simulink model "part_C_q17_simulink"  (R2023b)
settings: Solver=VariableStepAuto  StartTime=0.0  StopTime=20  RelTol=1e-3
values from neighbouring files (symbols this model uses):
  a1 = 1.4    [FOUND_full_car.m]
  a2 = 1.47    [FOUND_full_car.m]
  b1 = 0.7    [FOUND_full_car.m]
  b2 = 0.75    [FOUND_full_car.m]
  cf = 5000    [FOUND_full_car.m]
  cr = 5000    [FOUND_full_car.m]
  Ix = 820    [FOUND_full_car.m]
  Iy = 1100    [FOUND_full_car.m]
  kf = 10000    [FOUND_full_car.m]
  kr = 13000    [FOUND_full_car.m]
  ktf = 200000    [FOUND_full_car.m]
  ktr = 200000    [FOUND_full_car.m]
  m = 840    [FOUND_full_car.m]    (also in init_params.m = 240)
  mf = 53    [FOUND_full_car.m]
  mr = 76    [FOUND_full_car.m]
  w = b1+b2    (= 1.45)    [FOUND_full_car.m]    (also in q7.m = 2*pi*f; q8.m = 2*pi*f; roadpr_ISO8608.m = linspace(wmin,wmax,N)')
settings Model: Creator=yusufcagriogut  LastModifiedBy=yusufcagriogut

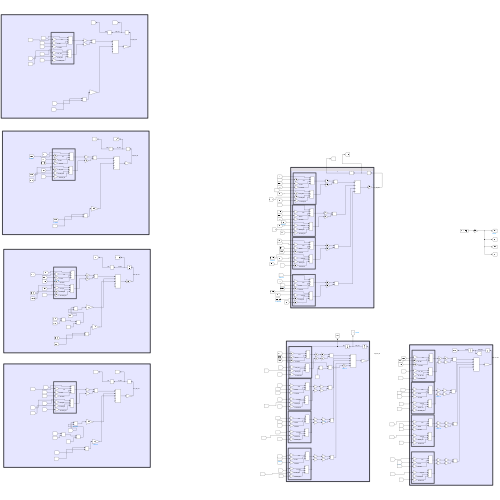
[thumbnail: Simulink's stored preview of the top-level diagram]
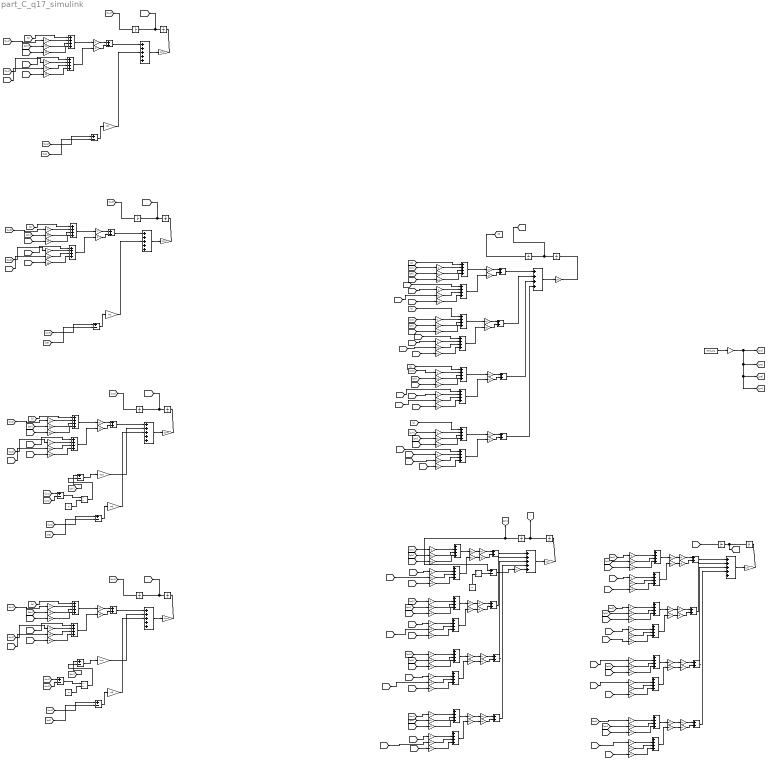
== system part_C_q17_simulink ==
  Add{,10..13,15..17,26,28..30,39,41,47,51} (16 alike) : Sum
  Add{1..9,18..25,31..38,43..46,49..50,53..54} (33 alike) : Sum  Inputs=++++
  Add{14,27,40,42,48,52} (6 alike) : Sum  Inputs=+++++
  Constant : Constant  Value=w
  Constant1 : Constant  Value=w
  Constant2 : Constant  Value=w
  Divide : Product  Inputs=*/
  Divide1 : Product  Inputs=*/
  Divide2 : Product  Inputs=*/
  From Workspace : FromWorkspace  VariableName=road_sig
  Gain : Gain  Gain=-kf
  Gain1 : Gain  Gain=-cf
  Gain{10,13,15,18,35,38,40,43,77,80,82,85,126,130,138,142} (16 alike) : Gain  Gain=-b2
  Gain{29,31,58,74,100} (5 alike) : Gain  Gain=-kr
  Gain{30,32,59,101} (4 alike) : Gain  Gain=-cr
  Gain{4,7,21,24,47,50,60,63,66..67,72..73,89,92,102,105,143,146,153,156} (20 alike) : Gain  Gain=b1
  Gain{5,8,11,14,36,39,61,64,78,81,103,106,127,131,144,147} (16 alike) : Gain  Gain=-a1
  Gain{3,6,9,12,17,20,23,26,37,42,46,49,52,56,62,65,79,84,88,91,94,98,104,107,125,129,137,139,141,145,152,155} (32 alike) : Gain  Gain=-1
  Gain{108..111} (4 alike) : Gain  Gain=a1
  Gain112 : Gain  Gain=-a2
  Gain113 : Gain  Gain=-a2
  Gain{16,19,22,25,41,44,48,51,83,86,90,93,114..115,140,148,154,157} (18 alike) : Gain  Gain=a2
  Gain{53,75,95,116,120} (5 alike) : Gain  Gain=kf
  Gain{54,76,96,117,121} (5 alike) : Gain  Gain=cf
  Gain118 : Gain  Gain=kr/w
  Gain119 : Gain  Gain=-ktf
  Gain122 : Gain  Gain=-kr/w
  Gain123 : Gain  Gain=-ktf
  Gain124 : Gain  Gain=1/mf
  Gain128 : Gain  Gain=1/mf
  Gain{55,97,132,134} (4 alike) : Gain  Gain=kr
  Gain{57,99,133,149} (4 alike) : Gain  Gain=cr
  Gain135 : Gain  Gain=-ktr
  Gain136 : Gain  Gain=1/mr
  Gain150 : Gain  Gain=-ktr
  Gain151 : Gain  Gain=1/mr
  Gain158 : Gain  Gain=0.01
  Gain2 : Gain  Gain=1/m
  Gain27 : Gain  Gain=-kf
  Gain28 : Gain  Gain=-cf
  Gain33 : Gain  Gain=-kf
  Gain34 : Gain  Gain=-cf
  Gain45 : Gain  Gain=1/Ix
  Gain{68..71} (4 alike) : Gain  Gain=b2
  Gain87 : Gain  Gain=1/Iy
  Integrator{,1..13} (14 alike) : Integrator
  Subtract{,1..7,9} (9 alike) : Sum  Inputs=+-
  wires:
  Gain/1 -> Add/1
  Gain1/1 -> Add/2
  Add/1 -> Add1/1
  Add1/1 -> Gain2/1
  Gain2/1 -> Integrator/1  "z_dot_dot"
  Add2/1 -> Gain/1
  Gain3/1 -> Add2/2  "-zu1"
  Gain4/1 -> Add2/3  "b1*phi"
  Gain5/1 -> Add2/4  "-a1*theta"
  Gain6/1 -> Add3/2  "-zu1_dot"
  Gain7/1 -> Add3/3  "b1*phi_dot"
  Gain8/1 -> Add3/4  "-a1*theta_dot"
  Add3/1 -> Gain1/1
  Gain14/1 -> Add5/4  "-a1*theta_dot"
  Gain13/1 -> Add5/3  "-b2*phi_dot"
  Gain12/1 -> Add5/2  "-zu2_dot"
  Gain11/1 -> Add4/4  "-a1*theta"
  Gain10/1 -> Add4/3  "-b2*phi"
  Gain9/1 -> Add4/2  "-zu2"
  Gain20/1 -> Add6/2  "-zu3"
  Gain15/1 -> Add6/3  "-b2*phi"
  Gain16/1 -> Add6/4  "a2*theta"
  Gain17/1 -> Add7/2  "-zu3_dot"
  Gain18/1 -> Add7/3  "-b2*phi_dot"
  Gain19/1 -> Add7/4  "a2*theta_dot"
  Gain21/1 -> Add8/3  "b1*phi"
  Gain25/1 -> Add9/4  "a2*theta_dot"
  Gain26/1 -> Add8/2  "-zu4"
  Gain24/1 -> Add9/3  "b1*phi_dot"
  Gain22/1 -> Add8/4  "a2*theta"
  Gain23/1 -> Add9/2  "-zu4_dot"
  Add5/1 -> Gain28/1
  Add4/1 -> Gain27/1
  Add10/1 -> Add1/2
  Gain28/1 -> Add10/2
  Gain27/1 -> Add10/1
  Gain29/1 -> Add11/1
  Gain30/1 -> Add11/2
  Add11/1 -> Add1/3
  Add6/1 -> Gain29/1
  Add7/1 -> Gain30/1
  Add9/1 -> Gain32/1
  Add8/1 -> Gain31/1
  Gain32/1 -> Add12/2
  Gain31/1 -> Add12/1
  Add12/1 -> Add1/4
  Add15/1 -> Add14/2
  Gain35/1 -> Add20/3  "-b2*phi"
  Add18/1 -> Gain66/1
  Gain58/1 -> Add17/1
  Add23/1 -> Gain70/1
  Gain59/1 -> Add17/2
  Gain62/1 -> Add19/2  "-zu1_dot"
  Gain34/1 -> Add13/2
  Add20/1 -> Gain68/1
  Add25/1 -> Gain73/1
  Add24/1 -> Gain72/1
  Gain57/1 -> Add16/2
  Gain45/1 -> Integrator2/1  "phi_dot_dot"
  Gain51/1 -> Add25/4  "a2*theta_dot"
  Gain56/1 -> Add18/2  "-zu1"
  Gain48/1 -> Add24/4  "a2*theta"
  Gain64/1 -> Add19/4  "-a1*theta_dot"
  Gain33/1 -> Add13/1
  Gain50/1 -> Add25/3  "b1*phi_dot"
  Add21/1 -> Gain69/1
  Gain36/1 -> Add20/4  "-a1*theta"
  Add17/1 -> Add14/4
  Gain38/1 -> Add21/3  "-b2*phi_dot"
  Add14/1 -> Gain45/1
  Gain52/1 -> Add24/2  "-zu4"
  Gain65/1 -> Add20/2  "-zu2"
  Gain49/1 -> Add25/2  "-zu4_dot"
  Gain40/1 -> Add22/3  "-b2*phi"
  Gain63/1 -> Add19/3  "b1*phi_dot"
  Gain60/1 -> Add18/3  "b1*phi"
  Gain47/1 -> Add24/3  "b1*phi"
  Integrator2/1 -> Integrator3/1, [phi_dot]  "phi_dot"
  Add22/1 -> Gain71/1
  Add19/1 -> Gain67/1
  Gain46/1 -> Add22/2  "-zu3"
  Gain61/1 -> Add18/4  "-a1*theta"
  Gain42/1 -> Add23/2  "-zu3_dot"
  Gain37/1 -> Add21/2  "-zu2_dot"
  Gain44/1 -> Add23/4  "a2*theta_dot"
  Add16/1 -> Add14/3
  Gain43/1 -> Add23/3  "-b2*phi_dot"
  Gain41/1 -> Add22/4  "a2*theta"
  Gain39/1 -> Add21/4  "-a1*theta_dot"
  Gain55/1 -> Add16/1
  Add13/1 -> Add14/1
  Gain53/1 -> Add15/1
  Gain54/1 -> Add15/2
  Gain66/1 -> Gain33/1
  Gain67/1 -> Gain34/1
  Integrator3/1 -> [phi], Subtract/1  "phi"
  Gain68/1 -> Gain53/1
  Gain69/1 -> Gain54/1
  Gain70/1 -> Gain57/1
  Gain71/1 -> Gain55/1
  Gain72/1 -> Gain58/1
  Gain73/1 -> Gain59/1
  Gain74/1 -> Add14/5
  Constant/1 -> Divide/2
  Divide/1 -> Subtract/2
  Subtract/1 -> Gain74/1
  Gain114/1 -> Gain100/1
  Gain113/1 -> Gain97/1
  Gain88/1 -> Add35/2  "-zu3"
  Add34/1 -> Gain111/1
  Gain81/1 -> Add34/4  "-a1*theta_dot"
  Gain112/1 -> Gain99/1
  Gain115/1 -> Gain101/1
  Add26/1 -> Add27/1
  Gain82/1 -> Add35/3  "-b2*phi"
  Gain90/1 -> Add37/4  "a2*theta"
  Gain110/1 -> Gain95/1
  Gain96/1 -> Add28/2
  Gain109/1 -> Gain76/1
  Add27/1 -> Gain87/1
  Gain106/1 -> Add32/4  "-a1*theta_dot"
  Gain99/1 -> Add29/2
  Gain87/1 -> Integrator4/1  "theta_dot_dot"
  Add29/1 -> Add27/3
  Gain111/1 -> Gain96/1
  Gain95/1 -> Add28/1
  Add36/1 -> Gain112/1
  Gain89/1 -> Add37/3  "b1*phi"
  Gain77/1 -> Add33/3  "-b2*phi"
  Gain108/1 -> Gain75/1
  Integrator4/1 -> [theta_dot], Integrator5/1  "theta_dot"
  Integrator1/1 -> [z]  "z"
  Gain105/1 -> Add32/3  "b1*phi_dot"
  Add32/1 -> Gain109/1
  Gain84/1 -> Add36/2  "-zu3_dot"
  Add37/1 -> Gain114/1
  Gain85/1 -> Add36/3  "-b2*phi_dot"
  Add35/1 -> Gain113/1
  Gain103/1 -> Add31/4  "-a1*theta"
  Gain79/1 -> Add34/2  "-zu2_dot"
  Add38/1 -> Gain115/1
  Gain97/1 -> Add29/1
  Gain86/1 -> Add36/4  "a2*theta_dot"
  Gain83/1 -> Add35/4  "a2*theta"
  Gain76/1 -> Add26/2
  Gain101/1 -> Add30/2
  Add31/1 -> Gain108/1
  Gain98/1 -> Add31/2  "-zu1"
  Add28/1 -> Add27/2
  Gain94/1 -> Add37/2  "-zu4"
  Gain104/1 -> Add32/2  "-zu1_dot"
  Add33/1 -> Gain110/1
  Gain100/1 -> Add30/1
  Gain93/1 -> Add38/4  "a2*theta_dot"
  Gain107/1 -> Add33/2  "-zu2"
  Gain92/1 -> Add38/3  "b1*phi_dot"
  Add30/1 -> Add27/4
  Gain102/1 -> Add31/3  "b1*phi"
  Gain80/1 -> Add34/3  "-b2*phi_dot"
  Gain78/1 -> Add33/4  "-a1*theta"
  Gain75/1 -> Add26/1
  Gain91/1 -> Add38/2  "-zu4_dot"
  Integrator/1 -> [z_dot], Integrator1/1
  [phi] -> Gain102/1
  Integrator5/1 -> [theta]  "theta"
  [theta] -> Gain103/1
  [theta_dot] -> Gain106/1
  [phi] -> Gain77/1
  [theta] -> Gain78/1
  [phi] -> Gain82/1
  [theta] -> Gain83/1
  [phi] -> Gain89/1
  [theta] -> Gain90/1
  [theta_dot] -> Gain81/1
  [theta_dot] -> Gain86/1
  [theta_dot] -> Gain93/1
  [theta_dot] -> Gain51/1
  [theta] -> Gain48/1
  [phi] -> Gain47/1
  [phi] -> Gain40/1
  [theta] -> Gain41/1
  [phi] -> Gain35/1
  [theta] -> Gain36/1
  [phi] -> Gain60/1
  [theta] -> Gain61/1
  [theta_dot] -> Gain64/1
  [theta_dot] -> Gain39/1
  [theta_dot] -> Gain44/1
  [theta_dot] -> Gain25/1
  [theta_dot] -> Gain19/1
  [theta_dot] -> Gain14/1
  [theta_dot] -> Gain8/1
  [phi] -> Gain4/1
  [theta] -> Gain5/1
  [phi] -> Gain10/1
  [theta] -> Gain11/1
  [phi] -> Gain15/1
  [theta] -> Gain16/1
  [phi] -> Gain21/1
  [theta] -> Gain22/1
  Add39/1 -> Add40/1
  Add45/1 -> Gain117/1
  Add40/1 -> Gain128/1
  Integrator7/1 -> [zu1]  "zu1"
  Gain128/1 -> Integrator6/1  "zu1_dot_dot"
  Add44/1 -> Gain116/1
  Integrator6/1 -> [zu1_dot], Integrator7/1  "zu1_dot"
  Gain144/1 -> Add44/4  "-a1*theta"
  Gain117/1 -> Add39/2
  Gain145/1 -> Add45/2  "-zu1_dot"
  Gain147/1 -> Add45/4  "-a1*theta_dot"
  Gain143/1 -> Add44/3  "b1*phi"
  Gain116/1 -> Add39/1
  [theta_dot] -> Gain147/1
  Gain146/1 -> Add45/3  "b1*phi_dot"
  [phi] -> Gain143/1
  [theta] -> Gain144/1
  Gain139/1 -> Add44/2  "-zu1"
  [z] -> Add44/1
  [zu1] -> Gain139/1
  [z_dot] -> Add45/1
  [zu1] -> Gain145/1
  [phi_dot] -> Gain146/1
  Gain118/1 -> Add40/2
  [phi] -> Subtract1/1
  Constant1/1 -> Divide1/2
  [zu1] -> Subtract2/1
  [zu2] -> Subtract2/2
  Subtract2/1 -> Divide1/1
  Divide1/1 -> Subtract1/2
  Subtract1/1 -> Gain118/1
  [zu1] -> Subtract3/1
  [zr1] -> Subtract3/2
  Subtract3/1 -> Gain119/1
  Gain119/1 -> Add40/3
  [zu2] -> Gain129/1
  Gain127/1 -> Add43/4  "-a1*theta"
  [zu2] -> Subtract5/2
  [zr2] -> Subtract6/2
  Add41/1 -> Add42/1
  Add42/1 -> Gain124/1
  Gain124/1 -> Integrator8/1  "zu2_dot_dot"
  Gain125/1 -> Add43/2  "-zu1"
  [theta] -> Gain127/1
  Integrator9/1 -> [zu2]  "zu2"
  Subtract4/1 -> Gain122/1
  [phi] -> Gain126/1
  Gain130/1 -> Add46/3  "b1*phi_dot"
  [theta_dot] -> Gain131/1
  Gain126/1 -> Add43/3  "b1*phi"
  Gain129/1 -> Add46/2  "-zu1_dot"
  Add43/1 -> Gain120/1
  Gain120/1 -> Add41/1
  Gain131/1 -> Add46/4  "-a1*theta_dot"
  Integrator8/1 -> [zu2_dot], Integrator9/1  "zu2_dot"
  Gain121/1 -> Add41/2
  [z_dot] -> Add46/1
  [phi_dot] -> Gain130/1
  [zu2] -> Gain125/1
  Constant2/1 -> Divide2/2
  [zu1] -> Subtract5/1
  [zu2] -> Subtract6/1
  Add46/1 -> Gain121/1
  Subtract5/1 -> Divide2/1
  Gain122/1 -> Add42/2
  Gain123/1 -> Add42/3
  Subtract6/1 -> Gain123/1
  Divide2/1 -> Subtract4/2
  [z] -> Add43/1
  [phi] -> Subtract4/1
  Add48/1 -> Gain136/1
  [phi_dot] -> Gain142/1
  [zr3] -> Subtract9/2
  [z] -> Add49/1
  Integrator10/1 -> [zu3_dot], Integrator11/1  "zu2_dot"
  Add49/1 -> Gain132/1
  Subtract9/1 -> Gain135/1
  [zu3] -> Subtract9/1
  Add50/1 -> Gain133/1
  [zu3] -> Gain137/1
  Gain132/1 -> Add47/1
  Gain133/1 -> Add47/2
  Gain142/1 -> Add50/3  "b1*phi_dot"
  [z_dot] -> Add50/1
  Gain140/1 -> Add49/4  "-a1*theta"
  Integrator11/1 -> [zu3]  "zu2"
  Gain135/1 -> Add48/3
  Gain137/1 -> Add49/2  "-zu1"
  [phi] -> Gain138/1
  [theta_dot] -> Gain148/1
  Gain136/1 -> Integrator10/1  "zu2_dot_dot"
  Gain148/1 -> Add50/4  "-a1*theta_dot"
  [theta] -> Gain140/1
  [zu3] -> Gain141/1
  Gain141/1 -> Add50/2  "-zu1_dot"
  Gain138/1 -> Add49/3  "b1*phi"
  Add47/1 -> Add48/1
  Gain134/1 -> Add51/1
  [zu4] -> Subtract7/1
  [phi_dot] -> Gain156/1
  Add51/1 -> Add52/1
  [z] -> Add53/1
  [theta] -> Gain154/1
  [z_dot] -> Add54/1
  [zr4] -> Subtract7/2
  Gain155/1 -> Add54/2  "-zu1_dot"
  Gain152/1 -> Add53/2  "-zu1"
  Gain150/1 -> Add52/3
  Add52/1 -> Gain151/1
  [zu4] -> Gain152/1
  Add53/1 -> Gain134/1
  Integrator12/1 -> [zu4_dot], Integrator13/1  "zu2_dot"
  Gain157/1 -> Add54/4  "-a1*theta_dot"
  [theta_dot] -> Gain157/1
  Gain154/1 -> Add53/4  "-a1*theta"
  Gain149/1 -> Add51/2
  Subtract7/1 -> Gain150/1
  [zu4] -> Gain155/1
  Add54/1 -> Gain149/1
  Gain156/1 -> Add54/3  "b1*phi_dot"
  [phi] -> Gain153/1
  Integrator13/1 -> [zu4]  "zu2"
  Gain151/1 -> Integrator12/1  "zu2_dot_dot"
  Gain153/1 -> Add53/3  "b1*phi"
  [zu1] -> Gain3/1
  [zu1_dot] -> Gain6/1
  [zu2] -> Gain9/1
  [zu2_dot] -> Gain12/1
  [zu3] -> Gain20/1
  [zu3_dot] -> Gain17/1
  [zu4] -> Gain26/1
  [zu4_dot] -> Gain23/1
  [zu1] -> Gain56/1
  [zu1_dot] -> Gain62/1
  [zu2] -> Gain65/1
  [zu2_dot] -> Gain37/1
  [zu3] -> Gain46/1
  [zu3_dot] -> Gain42/1
  [zu4] -> Gain52/1
  [zu4_dot] -> Gain49/1
  [zu1] -> Gain98/1
  [zu1_dot] -> Gain104/1
  [zu2] -> Gain107/1
  [zu2_dot] -> Gain79/1
  [zu2_dot] -> Gain88/1
  [zu3_dot] -> Gain84/1
  [zu4] -> Gain94/1
  [zu4_dot] -> Gain91/1
  From Workspace/1 -> Gain158/1
  [z] -> Add2/1
  [z_dot] -> Add3/1
  [phi_dot] -> Gain24/1
  [phi_dot] -> Gain18/1
  [phi_dot] -> Gain13/1
  [phi_dot] -> Gain7/1
  [phi_dot] -> Gain63/1
  [phi_dot] -> Gain38/1
  [phi_dot] -> Gain43/1
  [phi_dot] -> Gain50/1
  [z] -> Add4/1
  [z_dot] -> Add5/1
  [z] -> Add6/1
  [z_dot] -> Add7/1
  [z] -> Add8/1
  [z_dot] -> Add9/1
  Gain158/1 -> [zr4], [zr3], [zr2], [zr1]
